simulink model "TrayectoriasTesis"  (R2021b)
settings: Solver=ode45  StartTime=0.0  StopTime=200  MaxStep=0.1  RelTol=1e-3  EnableMultiTasking=on
settings Model: Creator=ceci  LastModifiedBy=fabia
settings SolverCC: AlgebraicLoopSolver=TrustRegion
settings DataIOCC: LimitDataPoints=on  SaveFormat=Array  ReturnWorkspaceOutputs=off
settings OptimizationCC: ExpressionDepthLimit=2147483647  LifeSpan=inf
settings DebuggingCC: UnderspecifiedInitializationDetection=Classic  MergeDetectMultiDrivingBlocksExec=none  SolverPrmCheckMsg=warning  StateNameClashWarn=warning  SFUnexpectedBacktrackingDiag=warning  SFNoUnconditionalDefaultTransitionDiag=warning  SFExecutionAtInitializationDiag=none  SFMachineParentedDataDiag=warning  ArithmeticOperatorsInVariantConditions=warning
settings HardwareCC: ProdBitPerPointer=32  ProdBitPerSizeT=32  ProdBitPerPtrDiffT=32  ProdLargestAtomicFloat=None  ProdIntDivRoundTo=Undefined  ProdEndianess=Unspecified  ProdWordSize=32  ProdHWDeviceType=32-bit Generic
settings ModelReferenceCC: PropagateSignalLabelsOutOfModel=off
settings SFSimCC: SimUseLocalCustomCode=off  CustomCodeUndefinedFunction=UseInterfaceOnly
settings RTWCC: RTWUseLocalCustomCode=off
settings CodeAppCC: StateflowObjectComments=on
settings GRTTargetCC: TargetLangStandard=C89/C90 (ANSI)
settings ConfigComp: CovMetricSettings=dw  CovSaveCumulativeToWorkspaceVar=on  CovSaveSingleToWorkspaceVar=on  CovExternalEMLEnable=off

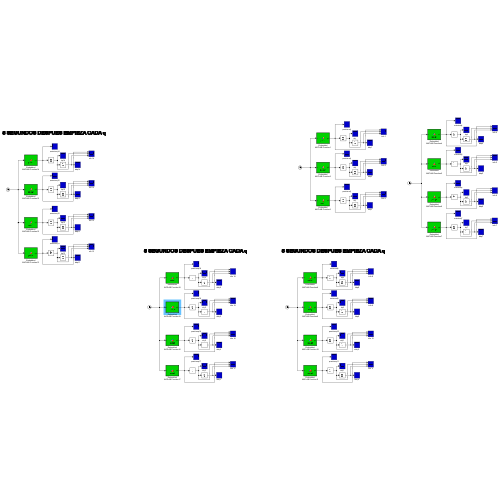
[thumbnail: Simulink's stored preview of the top-level diagram]
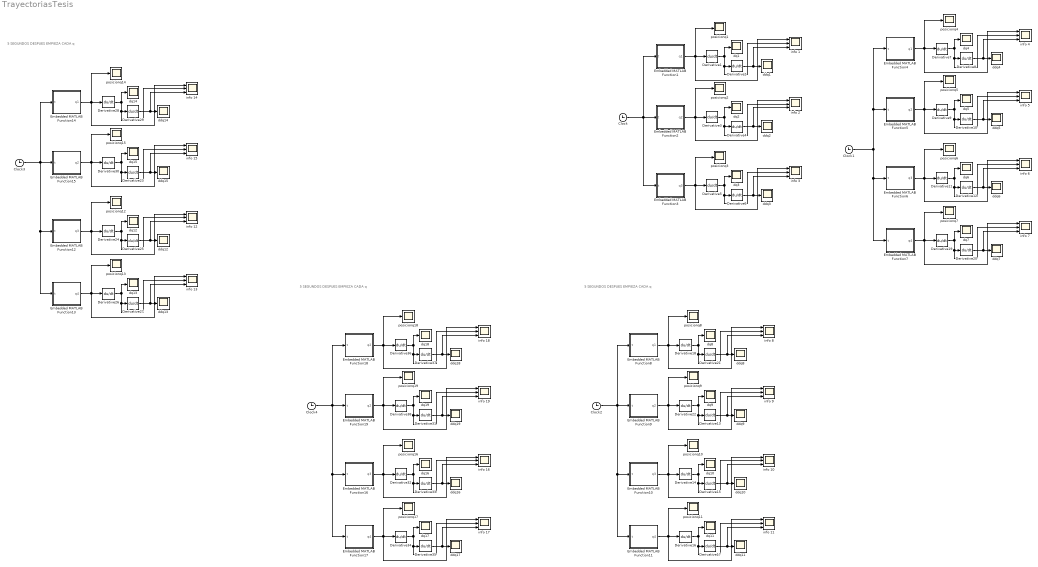
== system TrayectoriasTesis ==
  note: 5 SEGUNDOS DESPUES EMPIEZA CADA q
  note: 5 SEGUNDOS DESPUES EMPIEZA CADA q
  note: 5 SEGUNDOS DESPUES EMPIEZA CADA q
  Clock{,1..4} (5 alike) : Clock
      settings: Decimation=1000
  Derivative{1..38} (38 alike) : Derivative
  Embedded MATLAB Function1 : MATLAB Function  TreatAsAtomicUnit=on
  Embedded MATLAB Function10 : MATLAB Function  TreatAsAtomicUnit=on
  Embedded MATLAB Function11 : MATLAB Function  TreatAsAtomicUnit=on
  Embedded MATLAB Function12 : MATLAB Function  TreatAsAtomicUnit=on
  Embedded MATLAB Function13 : MATLAB Function  TreatAsAtomicUnit=on
  Embedded MATLAB Function14 : MATLAB Function  TreatAsAtomicUnit=on
  Embedded MATLAB Function15 : MATLAB Function  TreatAsAtomicUnit=on
  Embedded MATLAB Function16 : MATLAB Function  TreatAsAtomicUnit=on
  Embedded MATLAB Function17 : MATLAB Function  TreatAsAtomicUnit=on
  Embedded MATLAB Function18 : MATLAB Function  TreatAsAtomicUnit=on
  Embedded MATLAB Function19 : MATLAB Function  TreatAsAtomicUnit=on
  Embedded MATLAB Function2 : MATLAB Function  TreatAsAtomicUnit=on
  Embedded MATLAB Function3 : MATLAB Function  TreatAsAtomicUnit=on
  Embedded MATLAB Function4 : MATLAB Function  TreatAsAtomicUnit=on
  Embedded MATLAB Function5 : MATLAB Function  TreatAsAtomicUnit=on
  Embedded MATLAB Function6 : MATLAB Function  TreatAsAtomicUnit=on
  Embedded MATLAB Function7 : MATLAB Function  TreatAsAtomicUnit=on
  Embedded MATLAB Function8 : MATLAB Function  TreatAsAtomicUnit=on
  Embedded MATLAB Function9 : MATLAB Function  TreatAsAtomicUnit=on
  ddq{1..19} (19 alike) : Scope
  dq{1..19} (19 alike) : Scope
  info {1..19} (19 alike) : Scope  NumInputPorts=3
  posicionq{1..19} (19 alike) : Scope
  wires:
  Clock/1 -> Embedded MATLAB Function3/1(t), Embedded MATLAB Function2/1(t), Embedded MATLAB Function1/1(t)
  Embedded MATLAB Function1/1(q1) -> info 1/1, posicionq1/1, Derivative1/1
  Derivative2/1 -> info 1/3, ddq1/1
  Derivative1/1 -> info 1/2, Derivative2/1, dq1/1
  Embedded MATLAB Function2/1(q2) -> info 2/1, posicionq2/1, Derivative3/1
  Derivative4/1 -> info 2/3, ddq2/1
  Derivative3/1 -> info 2/2, Derivative4/1, dq2/1
  Embedded MATLAB Function3/1(q3) -> info 3/1, posicionq3/1, Derivative5/1
  Derivative6/1 -> info 3/3, ddq3/1
  Derivative5/1 -> info 3/2, Derivative6/1, dq3/1
  Derivative8/1 -> info 4/3, ddq4/1
  Derivative7/1 -> info 4/2, Derivative8/1, dq4/1
  Embedded MATLAB Function6/1(q3) -> info 6/1, posicionq6/1, Derivative11/1
  Embedded MATLAB Function5/1(q2) -> info 5/1, posicionq5/1, Derivative9/1
  Derivative9/1 -> info 5/2, Derivative10/1, dq5/1
  Derivative11/1 -> info 6/2, Derivative12/1, dq6/1
  Derivative12/1 -> info 6/3, ddq6/1
  Derivative10/1 -> info 5/3, ddq5/1
  Embedded MATLAB Function4/1(q1) -> info 4/1, posicionq4/1, Derivative7/1
  Clock1/1 -> Embedded MATLAB Function5/1(t), Embedded MATLAB Function4/1(t), Embedded MATLAB Function7/1(t), Embedded MATLAB Function6/1(t)
  Derivative19/1 -> info 7/2, Derivative20/1, dq7/1
  Derivative20/1 -> info 7/3, ddq7/1
  Embedded MATLAB Function7/1(q4) -> info 7/1, posicionq7/1, Derivative19/1
  Derivative17/1 -> info 11/3, ddq11/1
  Embedded MATLAB Function11/1(q4) -> info 11/1, posicionq11/1, Derivative16/1
  Derivative16/1 -> info 11/2, Derivative17/1, dq11/1
  Derivative15/1 -> info 10/3, ddq10/1
  Derivative14/1 -> info 10/2, Derivative15/1, dq10/1
  Derivative22/1 -> info 9/2, Derivative13/1, dq9/1
  Embedded MATLAB Function8/1(q1) -> info 8/1, posicionq8/1, Derivative18/1
  Derivative13/1 -> info 9/3, ddq9/1
  Clock2/1 -> Embedded MATLAB Function11/1(t), Embedded MATLAB Function10/1(t), Embedded MATLAB Function9/1(t), Embedded MATLAB Function8/1(t)
  Derivative21/1 -> info 8/3, ddq8/1
  Embedded MATLAB Function9/1(q2) -> info 9/1, posicionq9/1, Derivative22/1
  Derivative18/1 -> info 8/2, Derivative21/1, dq8/1
  Embedded MATLAB Function10/1(q3) -> info 10/1, posicionq10/1, Derivative14/1
  Derivative26/1 -> info 13/2, Derivative27/1, dq13/1
  Derivative24/1 -> info 12/2, Derivative25/1, dq12/1
  Derivative25/1 -> info 12/3, ddq12/1
  Embedded MATLAB Function13/1(q4) -> info 13/1, posicionq13/1, Derivative26/1
  Derivative28/1 -> info 14/2, Derivative29/1, dq14/1
  Embedded MATLAB Function15/1(q2) -> info 15/1, posicionq15/1, Derivative30/1
  Derivative27/1 -> info 13/3, ddq13/1
  Derivative29/1 -> info 14/3, ddq14/1
  Clock3/1 -> Embedded MATLAB Function13/1(t), Embedded MATLAB Function12/1(t), Embedded MATLAB Function15/1(t), Embedded MATLAB Function14/1(t)
  Derivative30/1 -> info 15/2, Derivative23/1, dq15/1
  Embedded MATLAB Function14/1(q1) -> info 14/1, posicionq14/1, Derivative28/1
  Derivative23/1 -> info 15/3, ddq15/1
  Embedded MATLAB Function12/1(q3) -> info 12/1, posicionq12/1, Derivative24/1
  Embedded MATLAB Function17/1(q4) -> info 17/1, posicionq17/1, Derivative34/1
  Derivative33/1 -> info 16/3, ddq16/1
  Derivative32/1 -> info 16/2, Derivative33/1, dq16/1
  Derivative35/1 -> info 17/3, ddq17/1
  Embedded MATLAB Function19/1(q2) -> info 19/1, posicionq19/1, Derivative38/1
  Derivative37/1 -> info 18/3, ddq18/1
  Embedded MATLAB Function16/1(q3) -> info 16/1, posicionq16/1, Derivative32/1
  Clock4/1 -> Embedded MATLAB Function17/1(t), Embedded MATLAB Function16/1(t), Embedded MATLAB Function19/1(t), Embedded MATLAB Function18/1(t)
  Embedded MATLAB Function18/1(q2) -> info 18/1, posicionq18/1, Derivative36/1
  Derivative38/1 -> info 19/2, Derivative31/1, dq19/1
  Derivative36/1 -> info 18/2, Derivative37/1, dq18/1
  Derivative34/1 -> info 17/2, Derivative35/1, dq17/1
  Derivative31/1 -> info 19/3, ddq19/1

== matlab function TrayectoriasTesis/Embedded MATLAB Function15 ==
  data: q2 output; t input
function q2 = posq2(t)
% This block supports an embeddable subset of the MATLAB language.
% See the help menu for details. 

if (t>=22)  % Si el t>=tmax, se repite una vez la rutina
    t=t-22;
end

if(t<8) % Movimiento 1
    t_inic = 0; % Tiempo en que inicia
    tf = 5;     % Tiempo en que termina
    y_ini = 0.785;
    y_f = -1.570;
elseif (t>=8 && t<16) % Movimiento 2
    t_inic = 8;
    tf = 5;
    y_ini =  -1.5706;
    y_f =  -1.570;
else  % Movimiento 3
    t_inic = 16;
    tf = 22;
    y_ini =  -1.570;
    y_f = 0.785;
end

% Calculo de trayectoria de tiempo minimo
Tb = tf/2;
% Vmax = 2*(y_f - y_ini)/(tf);
Vmax = (y_f - y_ini)/(tf - Tb);
ta = t - t_inic;
if(ta<0)
    q2 = y_ini;
elseif(ta >= 0 && ta < Tb)
    q2 = y_ini + (Vmax/(2*Tb))*ta*ta;
elseif(ta >= Tb && ta < (tf - Tb))
    q2 = (y_ini + y_f - Vmax*tf)/2 + Vmax*ta;
elseif(ta >= (tf - Tb) && ta < tf)
     q2 = y_f - (Vmax*(tf-ta)*(tf-ta)/(2*Tb));
else
    q2 = y_f;
end

== matlab function TrayectoriasTesis/Embedded MATLAB Function16 ==
  data: q3 output; t input
function q3 = posq3(t)
% This block supports an embeddable subset of the MATLAB language.
% See the help menu for details. 

if (t>=27)  % Si el t>=tmax, se repite una vez la rutina
    t=t-27;
end

if(t<16) % Movimiento 1
    t_inic = 10; % Tiempo en que inicia
    tf = 4;     % Tiempo en que termina
    y_ini = 1.570;
    y_f = -0.785;
elseif (t>=16 && t<22) % Movimiento 2
    t_inic = 16;
    tf = 4;
    y_ini = -0.785;
    y_f = -0.785;
else  % Movimiento 3
    t_inic = 22;
    tf = 5;
    y_ini = -0.785;
    y_f =  1.570;
end

% Calculo de trayectoria de tiempo minimo
Tb = tf/2;
% Vmax = 2*(y_f - y_ini)/(tf);
Vmax = (y_f - y_ini)/(tf - Tb);
ta = t - t_inic;
if(ta<0)
    q3 = y_ini;
elseif(ta >= 0 && ta < Tb)
    q3 = y_ini + (Vmax/(2*Tb))*ta*ta;
elseif(ta >= Tb && ta < (tf - Tb))
    q3 = (y_ini + y_f - Vmax*tf)/2 + Vmax*ta;
elseif(ta >= (tf - Tb) && ta < tf)
     q3 = y_f - (Vmax*(tf-ta)*(tf-ta)/(2*Tb));
else
    q3 = y_f;
end

== matlab function TrayectoriasTesis/Embedded MATLAB Function17 ==
  data: q4 output; t input
function q4 = posq4(t)

% This block supports an embeddable subset of the MATLAB language.
% See the help menu for details. 

if (t>=32)  % Si el t>=tmax, se repite una vez la rutina
    t=t-32;
end

if(t<12) % Movimiento 1
    t_inic = 0; % Tiempo en que inicia
    tf = 7;     % Tiempo en que termina
    y_ini = 3.14159;
    y_f = 0;
elseif (t>=12 && t<24) % Movimiento 2
    t_inic = 12;
    tf = 7;
    y_ini = 0;
    y_f = 0;
else  % Movimiento 3
    t_inic = 24;
    tf = 8;
    y_ini = 0;
    y_f = 3.14159;
end

% Calculo de trayectoria de tiempo minimo
Tb = tf/2;
% Vmax = 2*(y_f - y_ini)/(tf);
Vmax = (y_f - y_ini)/(tf - Tb);
ta = t - t_inic;
if(ta<0)
    q4 = y_ini;
elseif(ta >= 0 && ta < Tb)
    q4 = y_ini + (Vmax/(2*Tb))*ta*ta;
elseif(ta >= Tb && ta < (tf - Tb))
    q4 = (y_ini + y_f - Vmax*tf)/2 + Vmax*ta;
elseif(ta >= (tf - Tb) && ta < tf)
     q4 = y_f - (Vmax*(tf-ta)*(tf-ta)/(2*Tb));
else
    q4 = y_f;
end

== matlab function TrayectoriasTesis/Embedded MATLAB Function18 ==
  data: q2 output; t input
function q2 = posq2(t)
% This block supports an embeddable subset of the MATLAB language.
% See the help menu for details. 

if (t>=17)  % Si el t>=tmax, se repite una vez la rutina
    t=t-17;
end

if(t<6) % Movimiento 1
    t_inic = 0; % Tiempo en que inicia
    tf = 4;     % Tiempo en que termina
    y_ini = 0.785;
    y_f = -1.570;
elseif (t>=6 && t<12) % Movimiento 2
    t_inic = 6;
    tf = 4;
    y_ini =  -1.5706;
    y_f =  -1.570;
else  % Movimiento 3
    t_inic = 12;
    tf = 5;
    y_ini =  -1.570;
    y_f = 0.785;
end

% Calculo de trayectoria de tiempo minimo
Tb = tf/2;
% Vmax = 2*(y_f - y_ini)/(tf);
Vmax = (y_f - y_ini)/(tf - Tb);
ta = t - t_inic;
if(ta<0)
    q2 = y_ini;
elseif(ta >= 0 && ta < Tb)
    q2 = y_ini + (Vmax/(2*Tb))*ta*ta;
elseif(ta >= Tb && ta < (tf - Tb))
    q2 = (y_ini + y_f - Vmax*tf)/2 + Vmax*ta;
elseif(ta >= (tf - Tb) && ta < tf)
     q2 = y_f - (Vmax*(tf-ta)*(tf-ta)/(2*Tb));
else
    q2 = y_f;
end

== matlab function TrayectoriasTesis/Embedded MATLAB Function19 ==
  data: q2 output; t input
function q2 = posq2(t)
% This block supports an embeddable subset of the MATLAB language.
% See the help menu for details. 

if (t>=22)  % Si el t>=tmax, se repite una vez la rutina
    t=t-22;
end

if(t<11) % Movimiento 1
    t_inic = 5; % Tiempo en que inicia
    tf = 4;     % Tiempo en que termina
    y_ini = 0.785;
    y_f = -1.570;
elseif (t>=11 && t<17) % Movimiento 2
    t_inic = 11;
    tf = 4;
    y_ini =  -1.5706;
    y_f =  -1.570;
else  % Movimiento 3
    t_inic = 17;
    tf = 5;
    y_ini =  -1.570;
    y_f = 0.785;
end

% Calculo de trayectoria de tiempo minimo
Tb = tf/2;
% Vmax = 2*(y_f - y_ini)/(tf);
Vmax = (y_f - y_ini)/(tf - Tb);
ta = t - t_inic;
if(ta<0)
    q2 = y_ini;
elseif(ta >= 0 && ta < Tb)
    q2 = y_ini + (Vmax/(2*Tb))*ta*ta;
elseif(ta >= Tb && ta < (tf - Tb))
    q2 = (y_ini + y_f - Vmax*tf)/2 + Vmax*ta;
elseif(ta >= (tf - Tb) && ta < tf)
     q2 = y_f - (Vmax*(tf-ta)*(tf-ta)/(2*Tb));
else
    q2 = y_f;
end

== matlab function TrayectoriasTesis/Embedded MATLAB Function2 ==
  data: q2 output; t input
function q2 = posq2(t)
% This block supports an embeddable subset of the MATLAB language.
% See the help menu for details. 

if (t>=17)  % Si el t>=tmax, se repite una vez la rutina
    t=t-17;
end

if(t<6) % Movimiento 1
    t_inic = 0; % Tiempo en que inicia
    tf = 4;     % Tiempo en que termina
    y_ini = 1.570;
    y_f = -2.356
elseif (t>=6 && t<12) % Movimiento 2
    t_inic = 6;
    tf = 4;
    y_ini = -2.356;
    y_f = -2.356;
else  % Movimiento 3
    t_inic = 12;
    tf = 5;
    y_ini = -2.356;
    y_f = 0.785;
end

% Calculo de trayectoria de tiempo minimo
Tb = tf/2;
% Vmax = 2*(y_f - y_ini)/(tf);
Vmax = (y_f - y_ini)/(tf - Tb);
ta = t - t_inic;
if(ta<0)
    q2 = y_ini;
elseif(ta >= 0 && ta < Tb)
    q2 = y_ini + (Vmax/(2*Tb))*ta*ta;
elseif(ta >= Tb && ta < (tf - Tb))
    q2 = (y_ini + y_f - Vmax*tf)/2 + Vmax*ta;
elseif(ta >= (tf - Tb) && ta < tf)
     q2 = y_f - (Vmax*(tf-ta)*(tf-ta)/(2*Tb));
else
    q2 = y_f;
end

== matlab function TrayectoriasTesis/Embedded MATLAB Function3 ==
  data: q3 output; t input
function q3 = posq3(t)
% This block supports an embeddable subset of the MATLAB language.
% See the help menu for details. 

if (t>=17)  % Si el t>=tmax, se repite una vez la rutina
    t=t-17;
end

if(t<6) % Movimiento 1
    t_inic = 0; % Tiempo en que inicia
    tf = 4;     % Tiempo en que termina
    y_ini = 0.785;
    y_f = -1.570;
elseif (t>=6 && t<12) % Movimiento 2
    t_inic = 6;
    tf = 4;
    y_ini = -1.570;
    y_f = -3.14159;
else  % Movimiento 3
    t_inic = 12;
    tf = 5;
    y_ini = 3.14159;
    y_f = 0.785;
end

% Calculo de trayectoria de tiempo minimo
Tb = tf/2;
% Vmax = 2*(y_f - y_ini)/(tf);
Vmax = (y_f - y_ini)/(tf - Tb);
ta = t - t_inic;
if(ta<0)
    q3 = y_ini;
elseif(ta >= 0 && ta < Tb)
    q3 = y_ini + (Vmax/(2*Tb))*ta*ta;
elseif(ta >= Tb && ta < (tf - Tb))
    q3 = (y_ini + y_f - Vmax*tf)/2 + Vmax*ta;
elseif(ta >= (tf - Tb) && ta < tf)
     q3 = y_f - (Vmax*(tf-ta)*(tf-ta)/(2*Tb));
else
    q3 = y_f;
end

== matlab function TrayectoriasTesis/Embedded MATLAB Function4 ==
  data: q1 output; t input
function q1 = posq1(t)
% This block supports an embeddable subset of the MATLAB language.
% See the help menu for details. 

if (t>=17)  % Si el t>=tmax, se repite otra vez la rutina
    t=t-17;
end

if(t<6) % Movimiento 1
    t_inic = 0; % Tiempo en que inicia
    tf = 4;     % Tiempo en que termina
    y_ini = 0;  % Posicion articular inicial (rad)
    y_f = -3.14159;    % Posicion articular final (rad)
elseif (t>=6 && t<12) % Movimiento 2
    t_inic = 6;
    tf = 4;
    y_ini = -3.14159;
    y_f =-3.14159;
else  % Movimiento 3
    t_inic = 12;
    tf = 5;
    y_ini =-3.14159;
    y_f = 0;
end

% Calculo de trayectoria de tiempo minimo
Tb = tf/2;  % el tb queda a la mitad del tiempo final

% Vmax = 2*(y_f - y_ini)/(tf);

Vmax = (y_f - y_ini)/(tf - Tb);
ta = t - t_inic;

% Polinomios que describen la curva en funcion de tiempo
if(ta<0)
    q1 = y_ini;
elseif(ta >= 0 && ta < Tb)
    q1 = y_ini + (Vmax/(2*Tb))*ta*ta;
elseif(ta >= Tb && ta < (tf - Tb))
    q1 = (y_ini + y_f - Vmax*tf)/2 + Vmax*ta;
elseif(ta >= (tf - Tb) && ta < tf)
     q1 = y_f - (Vmax*(tf-ta)*(tf-ta)/(2*Tb));
else
    q1 = y_f;
end

== matlab function TrayectoriasTesis/Embedded MATLAB Function5 ==
  data: q2 output; t input
function q2 = posq2(t)
% This block supports an embeddable subset of the MATLAB language.
% See the help menu for details. 

if (t>=17)  % Si el t>=tmax, se repite una vez la rutina
    t=t-17;
end

if(t<6) % Movimiento 1
    t_inic = 0; % Tiempo en que inicia
    tf = 4;     % Tiempo en que termina
    y_ini = 0.785;
    y_f = -1.570;
elseif (t>=6 && t<12) % Movimiento 2
    t_inic = 6;
    tf = 4;
    y_ini =  -1.5706;
    y_f =  -1.570;
else  % Movimiento 3
    t_inic = 12;
    tf = 5;
    y_ini =  -1.570;
    y_f = 0.785;
end

% Calculo de trayectoria de tiempo minimo
Tb = tf/2;
% Vmax = 2*(y_f - y_ini)/(tf);
Vmax = (y_f - y_ini)/(tf - Tb);
ta = t - t_inic;
if(ta<0)
    q2 = y_ini;
elseif(ta >= 0 && ta < Tb)
    q2 = y_ini + (Vmax/(2*Tb))*ta*ta;
elseif(ta >= Tb && ta < (tf - Tb))
    q2 = (y_ini + y_f - Vmax*tf)/2 + Vmax*ta;
elseif(ta >= (tf - Tb) && ta < tf)
     q2 = y_f - (Vmax*(tf-ta)*(tf-ta)/(2*Tb));
else
    q2 = y_f;
end

== matlab function TrayectoriasTesis/Embedded MATLAB Function6 ==
  data: q3 output; t input
function q3 = posq3(t)
% This block supports an embeddable subset of the MATLAB language.
% See the help menu for details. 

if (t>=17)  % Si el t>=tmax, se repite una vez la rutina
    t=t-17;
end

if(t<6) % Movimiento 1
    t_inic = 0; % Tiempo en que inicia
    tf = 4;     % Tiempo en que termina
    y_ini = 1.570;
    y_f = -0.785;
elseif (t>=6 && t<12) % Movimiento 2
    t_inic = 6;
    tf = 4;
    y_ini = -0.785;
    y_f = -0.785;
else  % Movimiento 3
    t_inic = 12;
    tf = 5;
    y_ini = -0.785;
    y_f =  1.570;
end

% Calculo de trayectoria de tiempo minimo
Tb = tf/2;
% Vmax = 2*(y_f - y_ini)/(tf);
Vmax = (y_f - y_ini)/(tf - Tb);
ta = t - t_inic;
if(ta<0)
    q3 = y_ini;
elseif(ta >= 0 && ta < Tb)
    q3 = y_ini + (Vmax/(2*Tb))*ta*ta;
elseif(ta >= Tb && ta < (tf - Tb))
    q3 = (y_ini + y_f - Vmax*tf)/2 + Vmax*ta;
elseif(ta >= (tf - Tb) && ta < tf)
     q3 = y_f - (Vmax*(tf-ta)*(tf-ta)/(2*Tb));
else
    q3 = y_f;
end

== matlab function TrayectoriasTesis/Embedded MATLAB Function10 ==
  data: q3 output; t input
function q3 = posq3(t)
% This block supports an embeddable subset of the MATLAB language.
% See the help menu for details. 

if (t>=67)  % Si el t>=tmax, se repite una vez la rutina
    t=t-67;
end

if(t<26) % Movimiento 1
    t_inic = 0; % Tiempo en que inicia
    tf = 14;     % Tiempo en que termina
    y_ini = 1.570;
    y_f = -0.785;
elseif (t>=26 && t<52) % Movimiento 2
    t_inic = 26;
    tf = 14;
    y_ini = -0.785;
    y_f = -0.785;
else  % Movimiento 3
    t_inic = 52;
    tf = 15;
    y_ini = -0.785;
    y_f =  1.570;
end

% Calculo de trayectoria de tiempo minimo
Tb = tf/2;
% Vmax = 2*(y_f - y_ini)/(tf);
Vmax = (y_f - y_ini)/(tf - Tb);
ta = t - t_inic;
if(ta<0)
    q3 = y_ini;
elseif(ta >= 0 && ta < Tb)
    q3 = y_ini + (Vmax/(2*Tb))*ta*ta;
elseif(ta >= Tb && ta < (tf - Tb))
    q3 = (y_ini + y_f - Vmax*tf)/2 + Vmax*ta;
elseif(ta >= (tf - Tb) && ta < tf)
     q3 = y_f - (Vmax*(tf-ta)*(tf-ta)/(2*Tb));
else
    q3 = y_f;
end

== matlab function TrayectoriasTesis/Embedded MATLAB Function11 ==
  data: q4 output; t input
function q4 = posq4(t)

% This block supports an embeddable subset of the MATLAB language.
% See the help menu for details. 

if (t>=92)  % Si el t>=tmax, se repite una vez la rutina
    t=t-92;
end

if(t<36) % Movimiento 1
    t_inic = 0; % Tiempo en que inicia
    tf = 19;     % Tiempo en que termina
    y_ini = 3.14159;
    y_f = 0;
elseif (t>=36 && t<72) % Movimiento 2
    t_inic = 36;
    tf = 19;
    y_ini = 0;
    y_f = 0;
else  % Movimiento 3
    t_inic = 72;
    tf = 20;
    y_ini = 0;
    y_f = 3.14159;
end

% Calculo de trayectoria de tiempo minimo
Tb = tf/2;
% Vmax = 2*(y_f - y_ini)/(tf);
Vmax = (y_f - y_ini)/(tf - Tb);
ta = t - t_inic;
if(ta<0)
    q4 = y_ini;
elseif(ta >= 0 && ta < Tb)
    q4 = y_ini + (Vmax/(2*Tb))*ta*ta;
elseif(ta >= Tb && ta < (tf - Tb))
    q4 = (y_ini + y_f - Vmax*tf)/2 + Vmax*ta;
elseif(ta >= (tf - Tb) && ta < tf)
     q4 = y_f - (Vmax*(tf-ta)*(tf-ta)/(2*Tb));
else
    q4 = y_f;
end

== matlab function TrayectoriasTesis/Embedded MATLAB Function8 ==
  data: q1 output; t input
function q1 = posq1(t)
% This block supports an embeddable subset of the MATLAB language.
% See the help menu for details. 

if (t>=17)  % Si el t>=tmax, se repite otra vez la rutina
    t=t-17;
end

if(t<6) % Movimiento 1
    t_inic = 0; % Tiempo en que inicia
    tf = 4;     % Tiempo en que termina
    y_ini = 0;  % Posicion articular inicial (rad)
    y_f = -3.14159;    % Posicion articular final (rad)
elseif (t>=6 && t<12) % Movimiento 2
    t_inic = 6;
    tf = 4;
    y_ini = -3.14159;
    y_f =-3.14159;
else  % Movimiento 3
    t_inic = 12;
    tf = 5;
    y_ini =-3.14159;
    y_f = 0;
end

% Calculo de trayectoria de tiempo minimo
Tb = tf/2;  % el tb queda a la mitad del tiempo final

% Vmax = 2*(y_f - y_ini)/(tf);

Vmax = (y_f - y_ini)/(tf - Tb);
ta = t - t_inic;

% Polinomios que describen la curva en funcion de tiempo
if(ta<0)
    q1 = y_ini;
elseif(ta >= 0 && ta < Tb)
    q1 = y_ini + (Vmax/(2*Tb))*ta*ta;
elseif(ta >= Tb && ta < (tf - Tb))
    q1 = (y_ini + y_f - Vmax*tf)/2 + Vmax*ta;
elseif(ta >= (tf - Tb) && ta < tf)
     q1 = y_f - (Vmax*(tf-ta)*(tf-ta)/(2*Tb));
else
    q1 = y_f;
end

== matlab function TrayectoriasTesis/Embedded MATLAB Function7 ==
  data: q4 output; t input
function q4 = posq4(t)
% This block supports an embeddable subset of the MATLAB language.
% See the help menu for details. 

if (t>=17)  % Si el t>=tmax, se repite una vez la rutina
    t=t-17;
end

if(t<6) % Movimiento 1
    t_inic = 0; % Tiempo en que inicia
    tf = 4;     % Tiempo en que termina
    y_ini = 3.14159;
    y_f = 0;
elseif (t>=6 && t<12) % Movimiento 2
    t_inic = 6;
    tf = 4;
    y_ini = 0;
    y_f = 0;
else  % Movimiento 3
    t_inic = 12;
    tf = 5;
    y_ini = 0;
    y_f = 3.14159;
end

% Calculo de trayectoria de tiempo minimo
Tb = tf/2;
% Vmax = 2*(y_f - y_ini)/(tf);
Vmax = (y_f - y_ini)/(tf - Tb);
ta = t - t_inic;
if(ta<0)
    q4 = y_ini;
elseif(ta >= 0 && ta < Tb)
    q4 = y_ini + (Vmax/(2*Tb))*ta*ta;
elseif(ta >= Tb && ta < (tf - Tb))
    q4 = (y_ini + y_f - Vmax*tf)/2 + Vmax*ta;
elseif(ta >= (tf - Tb) && ta < tf)
     q4 = y_f - (Vmax*(tf-ta)*(tf-ta)/(2*Tb));
else
    q4 = y_f;
end

== matlab function TrayectoriasTesis/Embedded MATLAB Function9 ==
  data: q2 output; t input
function q2 = posq2(t)
% This block supports an embeddable subset of the MATLAB language.
% See the help menu for details. 

if (t>=42)  % Si el t>=tmax, se repite una vez la rutina
    t=t-42;
end

if(t<16) % Movimiento 1
    t_inic = 0; % Tiempo en que inicia
    tf = 9;     % Tiempo en que termina
    y_ini = 0.785;
    y_f = -1.570;
elseif (t>=16 && t<32) % Movimiento 2
    t_inic = 16;
    tf = 9;
    y_ini =  -1.5706;
    y_f =  -1.570;
else  % Movimiento 3
    t_inic = 32;
    tf = 10;
    y_ini =  -1.570;
    y_f = 0.785;
end

% Calculo de trayectoria de tiempo minimo
Tb = tf/2;
% Vmax = 2*(y_f - y_ini)/(tf);
Vmax = (y_f - y_ini)/(tf - Tb);
ta = t - t_inic;
if(ta<0)
    q2 = y_ini;
elseif(ta >= 0 && ta < Tb)
    q2 = y_ini + (Vmax/(2*Tb))*ta*ta;
elseif(ta >= Tb && ta < (tf - Tb))
    q2 = (y_ini + y_f - Vmax*tf)/2 + Vmax*ta;
elseif(ta >= (tf - Tb) && ta < tf)
     q2 = y_f - (Vmax*(tf-ta)*(tf-ta)/(2*Tb));
else
    q2 = y_f;
end

== matlab function TrayectoriasTesis/Embedded MATLAB Function1 ==
  data: q1 output; t input
function q1 = posq1(t)
% This block supports an embeddable subset of the MATLAB language.
% See the help menu for details. 

if (t>=17)  % Si el t>=tmax, se repite otra vez la rutina
    t=t-17;
end

if(t<6) % Movimiento 1
    t_inic = 0; % Tiempo en que inicia
    tf = 4;     % Tiempo en que termina
    y_ini = 0;  % Posicion articular inicial (rad)
    y_f = -3.14159;    % Posicion articular final (rad)
elseif (t>=6 && t<12) % Movimiento 2
    t_inic = 6;
    tf = 4;
    y_ini = -3.14159;
    y_f = -1.570;
else  % Movimiento 3
    t_inic = 12;
    tf = 5;
    y_ini = -1.570;
    y_f = 0;
end

% Calculo de trayectoria de tiempo minimo
Tb = tf/2;  % el tb queda a la mitad del tiempo final

% Vmax = 2*(y_f - y_ini)/(tf);

Vmax = (y_f - y_ini)/(tf - Tb);
ta = t - t_inic;

% Polinomios que describen la curva en funcion de tiempo
if(ta<0)
    q1 = y_ini;
elseif(ta >= 0 && ta < Tb)
    q1 = y_ini + (Vmax/(2*Tb))*ta*ta;
elseif(ta >= Tb && ta < (tf - Tb))
    q1 = (y_ini + y_f - Vmax*tf)/2 + Vmax*ta;
elseif(ta >= (tf - Tb) && ta < tf)
     q1 = y_f - (Vmax*(tf-ta)*(tf-ta)/(2*Tb));
else
    q1 = y_f;
end

== matlab function TrayectoriasTesis/Embedded MATLAB Function12 ==
  data: q3 output; t input
function q3 = posq3(t)
% This block supports an embeddable subset of the MATLAB language.
% See the help menu for details. 

if (t>=27)  % Si el t>=tmax, se repite una vez la rutina
    t=t-27;
end

if(t<10) % Movimiento 1
    t_inic = 0; % Tiempo en que inicia
    tf = 6;     % Tiempo en que termina
    y_ini = 1.570;
    y_f = -0.785;
elseif (t>=10 && t<20) % Movimiento 2
    t_inic = 10;
    tf = 16;
    y_ini = -0.785;
    y_f = -0.785;
else  % Movimiento 3
    t_inic = 20;
    tf = 7;
    y_ini = -0.785;
    y_f =  1.570;
end

% Calculo de trayectoria de tiempo minimo
Tb = tf/2;
% Vmax = 2*(y_f - y_ini)/(tf);
Vmax = (y_f - y_ini)/(tf - Tb);
ta = t - t_inic;
if(ta<0)
    q3 = y_ini;
elseif(ta >= 0 && ta < Tb)
    q3 = y_ini + (Vmax/(2*Tb))*ta*ta;
elseif(ta >= Tb && ta < (tf - Tb))
    q3 = (y_ini + y_f - Vmax*tf)/2 + Vmax*ta;
elseif(ta >= (tf - Tb) && ta < tf)
     q3 = y_f - (Vmax*(tf-ta)*(tf-ta)/(2*Tb));
else
    q3 = y_f;
end

== matlab function TrayectoriasTesis/Embedded MATLAB Function13 ==
  data: q4 output; t input
function q4 = posq4(t)

% This block supports an embeddable subset of the MATLAB language.
% See the help menu for details. 

if (t>=32)  % Si el t>=tmax, se repite una vez la rutina
    t=t-32;
end

if(t<12) % Movimiento 1
    t_inic = 0; % Tiempo en que inicia
    tf = 7;     % Tiempo en que termina
    y_ini = 3.14159;
    y_f = 0;
elseif (t>=12 && t<24) % Movimiento 2
    t_inic = 12;
    tf = 7;
    y_ini = 0;
    y_f = 0;
else  % Movimiento 3
    t_inic = 24;
    tf = 8;
    y_ini = 0;
    y_f = 3.14159;
end

% Calculo de trayectoria de tiempo minimo
Tb = tf/2;
% Vmax = 2*(y_f - y_ini)/(tf);
Vmax = (y_f - y_ini)/(tf - Tb);
ta = t - t_inic;
if(ta<0)
    q4 = y_ini;
elseif(ta >= 0 && ta < Tb)
    q4 = y_ini + (Vmax/(2*Tb))*ta*ta;
elseif(ta >= Tb && ta < (tf - Tb))
    q4 = (y_ini + y_f - Vmax*tf)/2 + Vmax*ta;
elseif(ta >= (tf - Tb) && ta < tf)
     q4 = y_f - (Vmax*(tf-ta)*(tf-ta)/(2*Tb));
else
    q4 = y_f;
end

== matlab function TrayectoriasTesis/Embedded MATLAB Function14 ==
  data: q1 output; t input
function q1 = posq1(t)
% This block supports an embeddable subset of the MATLAB language.
% See the help menu for details. 

if (t>=17)  % Si el t>=tmax, se repite otra vez la rutina
    t=t-17;
end

if(t<6) % Movimiento 1
    t_inic = 0; % Tiempo en que inicia
    tf = 4;     % Tiempo en que termina
    y_ini = 0;  % Posicion articular inicial (rad)
    y_f = -3.14159;    % Posicion articular final (rad)
elseif (t>=6 && t<12) % Movimiento 2
    t_inic = 6;
    tf = 4;
    y_ini = -3.14159;
    y_f =-3.14159;
else  % Movimiento 3
    t_inic = 12;
    tf = 5;
    y_ini =-3.14159;
    y_f = 0;
end

% Calculo de trayectoria de tiempo minimo
Tb = tf/2;  % el tb queda a la mitad del tiempo final

% Vmax = 2*(y_f - y_ini)/(tf);

Vmax = (y_f - y_ini)/(tf - Tb);
ta = t - t_inic;

% Polinomios que describen la curva en funcion de tiempo
if(ta<0)
    q1 = y_ini;
elseif(ta >= 0 && ta < Tb)
    q1 = y_ini + (Vmax/(2*Tb))*ta*ta;
elseif(ta >= Tb && ta < (tf - Tb))
    q1 = (y_ini + y_f - Vmax*tf)/2 + Vmax*ta;
elseif(ta >= (tf - Tb) && ta < tf)
     q1 = y_f - (Vmax*(tf-ta)*(tf-ta)/(2*Tb));
else
    q1 = y_f;
end
